simulink model "VirtualDAQ"  (R2021b)
settings: Solver=VariableStepAuto  StartTime=0.0  StopTime=inf  MaxStep=0.001  RelTol=1e-3
libraries: fl_lib x5, simulink x3, nesl_utility x3, dspxfrm3 x1
(part 2 of 2)

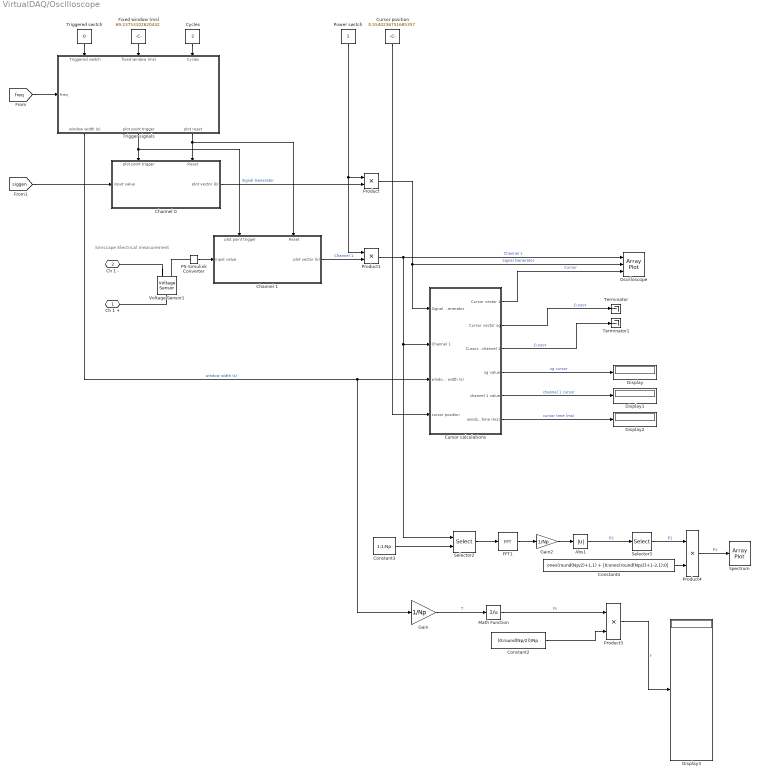
== system VirtualDAQ/Oscilloscope ==
  note: Simscape Electrical measurement
  Abs1 : Abs
  Channel 0 : Subsystem
      settings: PortSchema="{\"entries\":[{\"content\":{\"sides\":[{\"content\":{\"connectorIds\":[\"In1\"]},\"type\":\"ConnectorPlacement.EquallySpacedRectSide\",\"uuid\":\"56eea059-d5e9-4d95-b7d9-83a317b3103e\"},{\"content\":{\"connectorIds\":[\"Out1\"],\"side\":\"RIGHT\"},\"type\":\"ConnectorPlacement.EquallySpacedRectSide\",\"uuid\":\"fd8b8cd5-6def-4d8f-87ca-646372cc7fbe\"},{\"content\":{\"connectorIds\":[\"In2\",\"In3\"],\"side\":\"TOP\"},\"type\":\"ConnectorPlacement.EquallySpacedRectSide\",\"uuid\":\"3d9c38ee-b24b-466c-a7ac-a6d8a7456d51\"},{\"content\":{\"connectorIds\":[],\"side\":\"BOTTOM\"},\"type\":\"ConnectorPlacement.EquallySpacedRectSide\",\"uuid\":\"336136fa-2514-49ab-9e17-88caaca7366c\"}]},\"type\":\"ConnectorPlacement.EquallySpacedConnector\",\"uuid\":\"1d9824a8-6efd-49ff-b082-cf2ede19b4fd\"}],\"packageUris\":[\"http://schema.mathworks.com/mf0/Connector/R2020b\"],\"version\":\"1.0\"}"
  Channel 1 : Subsystem
      settings: PortSchema="{\"entries\":[{\"content\":{\"sides\":[{\"content\":{\"connectorIds\":[\"In1\"]},\"type\":\"ConnectorPlacement.EquallySpacedRectSide\",\"uuid\":\"56eea059-d5e9-4d95-b7d9-83a317b3103e\"},{\"content\":{\"connectorIds\":[\"Out1\"],\"side\":\"RIGHT\"},\"type\":\"ConnectorPlacement.EquallySpacedRectSide\",\"uuid\":\"fd8b8cd5-6def-4d8f-87ca-646372cc7fbe\"},{\"content\":{\"connectorIds\":[\"In2\",\"In3\"],\"side\":\"TOP\"},\"type\":\"ConnectorPlacement.EquallySpacedRectSide\",\"uuid\":\"3d9c38ee-b24b-466c-a7ac-a6d8a7456d51\"},{\"content\":{\"connectorIds\":[],\"side\":\"BOTTOM\"},\"type\":\"ConnectorPlacement.EquallySpacedRectSide\",\"uuid\":\"336136fa-2514-49ab-9e17-88caaca7366c\"}]},\"type\":\"ConnectorPlacement.EquallySpacedConnector\",\"uuid\":\"1d9824a8-6efd-49ff-b082-cf2ede19b4fd\"}],\"packageUris\":[\"http://schema.mathworks.com/mf0/Connector/R2020b\"],\"version\":\"1.0\"}"
  Constant2 : Constant  Value=(0:round(Np/2))/Np
  Constant3 : Constant  Value=1:1:Np
  Constant4 : Constant  Value=ones(round(Np/2)+1,1) + [0;ones(round(Np/2)+1-2,1);0]
  Cursor calculations : Subsystem
  Cursor position : Constant  Value=0.5540236751685357
  Cycles : Constant  Value=2
  Display{,1..3} (4 alike) : Display
  FFT1 : dspxfrm3/FFT  FFTImplementation=Auto  CompMethod=Table lookup  TableOpt=NEW  TableOptActive=Speed  BitRevOrder=off  Normalize=off  InheritFFTLength=on  FFTLength=64  WrapInput=on  roundingMode=Floor  overflowMode=off  firstCoeffDataTypeStr=Inherit: Same word length as input  firstCoeffLastDataTypeStr=Inherit: Same word length as input  outputMin=[]  outputMax=[]
  Fixed window (ms) : Constant  Value=69.23753102620442
  Gain : Gain  Gain=1/Np
  Gain2 : Gain  Gain=1/Np
  Math Function : Math  Operator=reciprocal  SaturateOnIntegerOverflow=on
  Oscilloscope : ArrayPlot  NumInputPorts=3  WindowPosition=[1282.000000,742.000000,1279.000000,669.000000,]  Visible=on  PlotType=Line  AxesScaling=Manual  YLimits=[-5.1,5.1]  ShowLegend=on
  PS-Simulink Converter : nesl_utility/PS-Simulink Converter  PhysicalDomain=network_engine_domain  SubClassName=ps_output  LeftPortType=input  RightPortType=output  PseudoPeriodic=off  Frequencies=[]  Unit=inherit  AffineConversion=off
      settings: SourceProductBaseCode=PW,SS
  Power switch : Constant
  Product{,1,3..4} (4 alike) : Product
  Selector2 : Selector  InputPortWidth=Np  IndexOptions=Index vector (port)  Indices=1:4:Np  OutputSizes=1
  Selector3 : Selector  InputPortWidth=Np  IndexOptions=Index vector (dialog)  Indices=1:round(Np/2)+1  OutputSizes=1
  Spectrum : ArrayPlot  WindowPosition=[1282.000000,42.000000,1279.000000,669.000000,]  Visible=on  YLimits=[-0.20978091343649902,1.9504387414806172]
  Terminator : Terminator
  Terminator1 : Terminator
  Trigger signals : Subsystem
      settings: PortSchema="{\"entries\":[{\"content\":{\"sides\":[{\"content\":{\"connectorIds\":[\"In1\"]},\"type\":\"ConnectorPlacement.EquallySpacedRectSide\",\"uuid\":\"b92255b7-066e-487b-9e0c-e19692fc940f\"},{\"content\":{\"connectorIds\":[],\"side\":\"RIGHT\"},\"type\":\"ConnectorPlacement.EquallySpacedRectSide\",\"uuid\":\"cb964d42-f40b-466c-b45b-853437324272\"},{\"content\":{\"connectorIds\":[\"In2\",\"In3\",\"In4\"],\"side\":\"TOP\"},\"type\":\"ConnectorPlacement.EquallySpacedRectSide\",\"uuid\":\"e1027385-b295-47a3-ae7d-2e3bb07fa1de\"},{\"content\":{\"connectorIds\":[\"Out1\",\"Out2\",\"Out3\"],\"side\":\"BOTTOM\"},\"type\":\"ConnectorPlacement.EquallySpacedRectSide\",\"uuid\":\"c27dc584-c0ba-4e72-b8bf-7374d1985911\"}]},\"type\":\"ConnectorPlacement.EquallySpacedConnector\",\"uuid\":\"1db11e79-2cf0-4841-86d9-651820ebc8ee\"}],\"packageUris\":[\"http://schema.mathworks.com/mf0/Connector/R2020b\"],\"version\":\"1.0\"}"
  Triggered switch : Constant  Value=0
  Voltage Sensor1 : fl_lib/Electrical/Electrical Sensors/Voltage Sensor
  Ch 1 + : PMIOPort  Side=Right
  Ch 1 - : PMIOPort  Port=2  Side=Right
  wires:
  PS-Simulink Converter/1 -> Channel 1/1(input value)
  Trigger signals/3("plot reset ") -> Channel 0/3(Reset), Channel 1/3(Reset)
  Trigger signals/2(plot point trigger) -> Channel 0/2(plot point trigger), Channel 1/2(plot point trigger)
  [freq] -> Trigger signals/1(freq)
  Product/1 -> Oscilloscope/2, Cursor calculations/1(Signal Generator)  "Signal Generator"
  [siggen] -> Channel 0/1(input value)
  Power switch/1 -> Product1/1, Product/1
  Channel 0/1(plot vector (k)) -> Product/2  "Signal Generator"
  Channel 1/1(plot vector (k)) -> Product1/2  "Channel 1"
  Triggered switch/1 -> Trigger signals/2(Triggered switch)
  Cycles/1 -> Trigger signals/4(Cycles)
  Cursor position/1 -> Cursor calculations/4(cursor position)
  Cursor calculations/1(Cursor vector 1) -> Oscilloscope/3  "Cursor"
  Cursor calculations/4(sg value) -> Display/1  "sg cursor"
  Cursor calculations/5(channel 1 value) -> Display1/1  "channel 1 cursor"
  Cursor calculations/3(Cursor vector channel 1) -> Terminator1/1  "Cursor"
  Cursor calculations/6(window time (ms)) -> Display2/1  "cursor time (ms)"
  Cursor calculations/2(Cursor vector sg) -> Terminator/1  "Cursor"
  Trigger signals/1(window width (s)) -> Gain/1, Cursor calculations/3(window width (s))  "window width (s)"
  Fixed window (ms)/1 -> Trigger signals/3(fixed window (ms))
  Gain/1 -> Math Function/1  "T"
  Math Function/1 -> Product3/1  "Fs"
  Constant2/1 -> Product3/2
  Product3/1 -> Display3/1  "f"
  Constant4/1 -> Product4/2
  FFT1/1 -> Gain2/1
  Constant3/1 -> Selector2/2
  Product4/1 -> Spectrum/1  "P1"
  Product1/1 -> Cursor calculations/2(Channel 1), Selector2/1, Oscilloscope/1  "Channel 1"
  Selector2/1 -> FFT1/1
  Gain2/1 -> Abs1/1
  Selector3/1 -> Product4/1  "P1"
  Abs1/1 -> Selector3/1  "P2"
  connections:
  Voltage Sensor1/RConn2 -- Ch 1 -/RConn1
  Voltage Sensor1/RConn1 -- PS-Simulink Converter/LConn1
  Voltage Sensor1/LConn1 -- Ch 1 +/RConn1

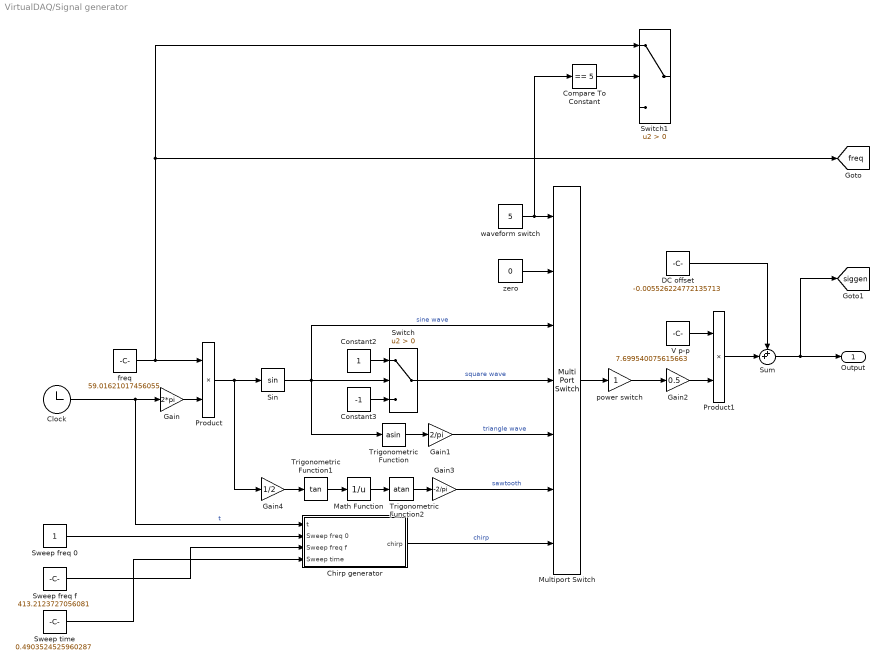
== system VirtualDAQ/Signal generator ==
  Chirp generator : Subsystem
  Clock : Clock
  Compare To Constant : simulink/Logic and Bit Operations/Compare To Constant  relop===  const=5  OutDataTypeStr=boolean
  Constant2 : Constant  SampleTime=0
  Constant3 : Constant  Value=-1  SampleTime=0
  DC offset : Constant  Value=-0.005526224772135713
  Gain : Gain  Gain=2*pi
  Gain1 : Gain  Gain=2/pi
  Gain2 : Gain  Gain=0.5
  Gain3 : Gain  Gain=-2/pi
  Gain4 : Gain  Gain=1/2
  Math Function : Math  Operator=reciprocal  SaturateOnIntegerOverflow=on
  Multiport Switch : MultiPortSwitch  DataPortOrder=Zero-based contiguous  Inputs=6  DiagnosticForDefault=None  zeroidx=on
  Product : Product
  Product1 : Product
  Sin : Trigonometry
  Sum : Sum  Inputs=++|
  Sweep freq 0 : Constant
  Sweep freq f : Constant  Value=413.2123727056081
  Sweep time : Constant  Value=0.4903524525960287
  Switch : Switch  Criteria=u2 > Threshold
  Switch1 : Switch  Criteria=u2 > Threshold
  Trigonometric Function : Trigonometry  Operator=asin
  Trigonometric Function1 : Trigonometry  Operator=tan
  Trigonometric Function2 : Trigonometry  Operator=atan
  V p-p : Constant  Value=7.699540075615663  SampleTime=-1
  freq : Constant  Value=59.01621017456055  SampleTime=0
  power switch : Gain
  waveform switch : Constant  Value=5  SampleTime=0
  zero : Constant  Value=0  SampleTime=0
  Output : Outport
  tag scope: freq=global, siggen=global
  wires:
  Sin/1 -> Trigonometric Function/1, Multiport Switch/3, Switch/2  "sine wave"
  freq/1 -> Switch1/1, [freq], Product/1
  Clock/1 -> Chirp generator/1(t), Gain/1  "t"
  power switch/1 -> Gain2/1
  zero/1 -> Multiport Switch/2
  Trigonometric Function/1 -> Gain1/1
  Constant2/1 -> Switch/1
  Constant3/1 -> Switch/3
  Gain2/1 -> Product1/2
  Product/1 -> Sin/1, Gain4/1
  Gain1/1 -> Multiport Switch/5  "triangle wave"
  Math Function/1 -> Trigonometric Function2/1
  Trigonometric Function1/1 -> Math Function/1
  Trigonometric Function2/1 -> Gain3/1
  Gain4/1 -> Trigonometric Function1/1
  Multiport Switch/1 -> power switch/1
  Gain3/1 -> Multiport Switch/6  "sawtooth"
  V p-p/1 -> Product1/1
  Product1/1 -> Sum/2
  DC offset/1 -> Sum/1
  Switch/1 -> Multiport Switch/4  "square wave"
  Sum/1 -> [siggen], Output/1
  Gain/1 -> Product/2
  Sweep time/1 -> Chirp generator/4(Sweep time)
  Chirp generator/1(chirp) -> Multiport Switch/7  "chirp"
  Sweep freq 0/1 -> Chirp generator/2(Sweep freq 0)
  Sweep freq f/1 -> Chirp generator/3(Sweep freq f)
  Compare To Constant/1 -> Switch1/2
  waveform switch/1 -> Compare To Constant/1, Multiport Switch/1

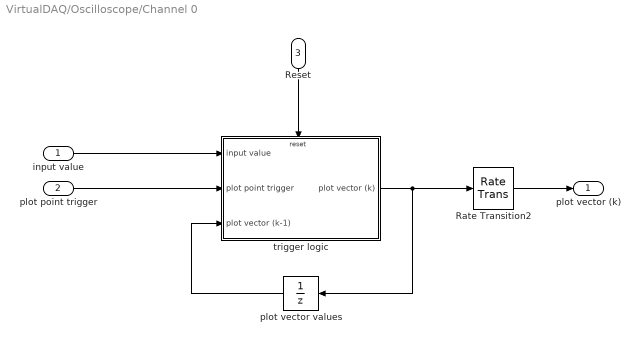
== system VirtualDAQ/Oscilloscope/Channel 0 ==
  input value : Inport
  plot point trigger : Inport  Port=2
  Reset : Inport  Port=3
  Rate Transition2 : RateTransition  InitialCondition=zeros(Np,1)  OutPortSampleTime=1/refreshRate
  plot vector values : UnitDelay  InitialCondition=zeros(Np,1)  SampleTime=-1  HasFrameUpgradeWarning=on
  trigger logic : Subsystem  TreatAsAtomicUnit=on
  plot vector (k) : Outport
  wires:
  plot vector values/1 -> trigger logic/3(plot vector (k-1))
  plot point trigger/1 -> trigger logic/2(plot point trigger)
  trigger logic/1(plot vector (k)) -> Rate Transition2/1, plot vector values/1
  Reset/1 -> trigger logic/Reset
  input value/1 -> trigger logic/1(input value)
  Rate Transition2/1 -> plot vector (k)/1

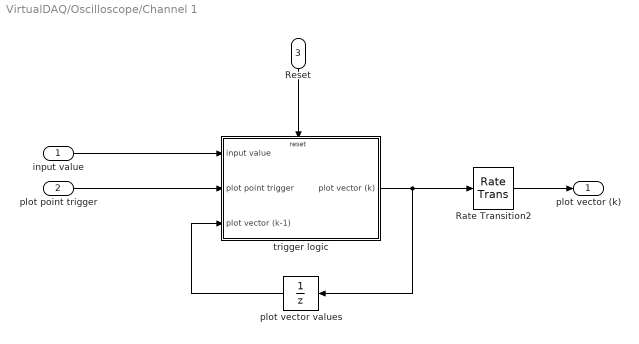
== system VirtualDAQ/Oscilloscope/Channel 1 ==
  input value : Inport
  plot point trigger : Inport  Port=2
  Reset : Inport  Port=3
  Rate Transition2 : RateTransition  InitialCondition=zeros(Np,1)  OutPortSampleTime=1/refreshRate
  plot vector values : UnitDelay  InitialCondition=zeros(Np,1)  SampleTime=-1  HasFrameUpgradeWarning=on
  trigger logic : Subsystem  TreatAsAtomicUnit=on
  plot vector (k) : Outport
  wires:
  plot vector values/1 -> trigger logic/3(plot vector (k-1))
  plot point trigger/1 -> trigger logic/2(plot point trigger)
  trigger logic/1(plot vector (k)) -> Rate Transition2/1, plot vector values/1
  Reset/1 -> trigger logic/Reset
  input value/1 -> trigger logic/1(input value)
  Rate Transition2/1 -> plot vector (k)/1

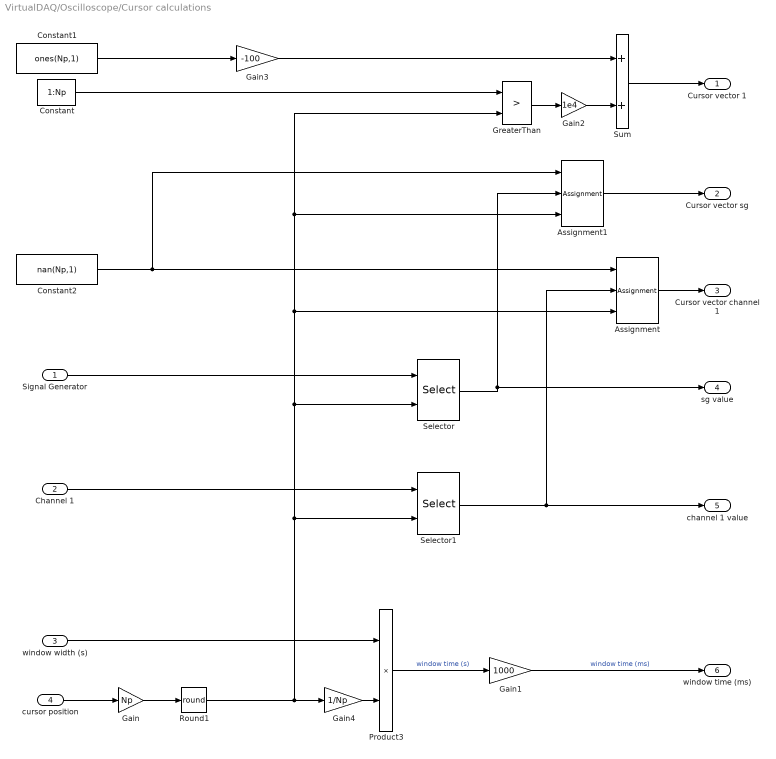
== system VirtualDAQ/Oscilloscope/Cursor calculations ==
  Signal Generator : Inport
  Channel 1 : Inport  Port=2
  window width (s) : Inport  Port=3
  cursor position : Inport  Port=4
  Assignment : Assignment  DiagnosticForDimensions=Warning  IndexOptions=Index vector (port)  Indices=1  OutputSizes=1
  Assignment1 : Assignment  DiagnosticForDimensions=Warning  IndexOptions=Index vector (port)  Indices=1  OutputSizes=1
  Constant : Constant  Value=1:Np
  Constant1 : Constant  Value=ones(Np,1)
  Constant2 : Constant  Value=nan(Np,1)
  Gain : Gain  Gain=Np
  Gain1 : Gain  Gain=1000
  Gain2 : Gain  Gain=1e4
  Gain3 : Gain  Gain=-100
  Gain4 : Gain  Gain=1/Np
  GreaterThan : RelationalOperator  Operator=>  OutDataTypeStr=boolean  RndMeth=Simplest
  Product3 : Product
  Round1 : Rounding  Operator=round
  Selector : Selector  InputPortWidth=Np  IndexOptions=Index vector (port)  Indices=[1 3]  OutputSizes=1
  Selector1 : Selector  InputPortWidth=Np  IndexOptions=Index vector (port)  Indices=[1 3]  OutputSizes=1
  Sum : Sum
  Cursor vector 1 : Outport
  Cursor vector sg : Outport  Port=2
  Cursor vector channel 1 : Outport  Port=3
  sg value : Outport  Port=4
  channel 1 value : Outport  Port=5
  window time (ms) : Outport  Port=6
  wires:
  cursor position/1 -> Gain/1
  Constant/1 -> GreaterThan/1
  Product3/1 -> Gain1/1  "window time (s)"
  Gain1/1 -> window time (ms)/1  "window time (ms)"
  GreaterThan/1 -> Gain2/1
  Sum/1 -> Cursor vector 1/1
  Gain2/1 -> Sum/2
  Signal Generator/1 -> Selector/1
  Selector1/1 -> Assignment/2, channel 1 value/1
  Constant1/1 -> Gain3/1
  Gain3/1 -> Sum/1
  Gain/1 -> Round1/1
  Gain4/1 -> Product3/2
  Channel 1/1 -> Selector1/1
  Assignment/1 -> Cursor vector channel 1/1
  Selector/1 -> Assignment1/2, sg value/1
  Round1/1 -> Selector/2, Assignment1/3, GreaterThan/2, Assignment/3, Selector1/2, Gain4/1
  Assignment1/1 -> Cursor vector sg/1
  Constant2/1 -> Assignment1/1, Assignment/1
  window width (s)/1 -> Product3/1

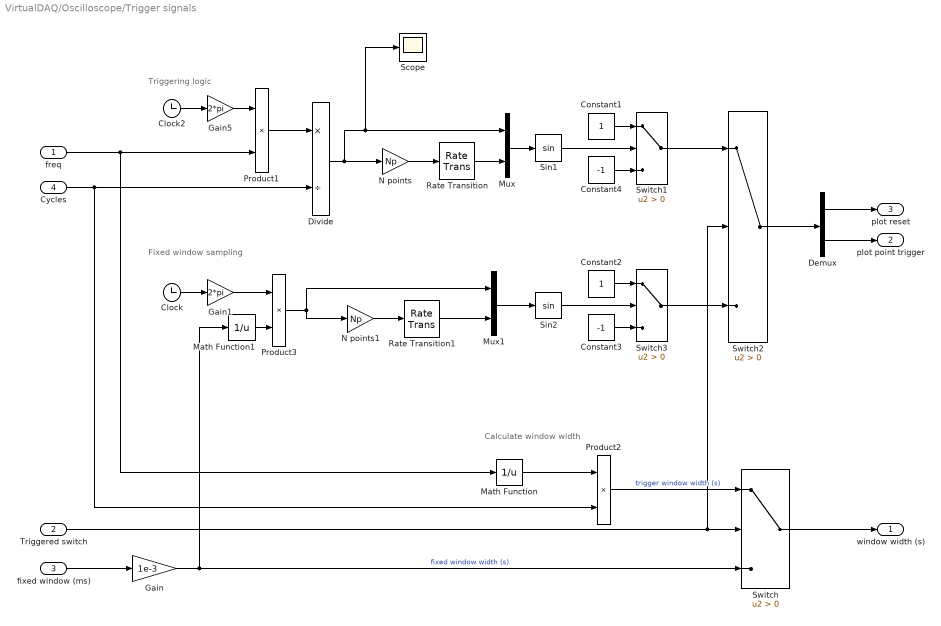
== system VirtualDAQ/Oscilloscope/Trigger signals ==
  note: Calculate window width
  note: Triggering logic
  note: Fixed window sampling
  freq : Inport
  Triggered switch : Inport  Port=2
  fixed window (ms) : Inport  Port=3
  Cycles : Inport  Port=4
  Clock : Clock
  Clock2 : Clock
  Constant1 : Constant  SampleTime=0
  Constant2 : Constant  SampleTime=0
  Constant3 : Constant  Value=-1  SampleTime=0
  Constant4 : Constant  Value=-1  SampleTime=0
  Demux : Demux  Outputs=2
  Divide : Product  Inputs=*/
  Gain : Gain  Gain=1e-3
  Gain1 : Gain  Gain=2*pi
  Gain5 : Gain  Gain=2*pi
  Math Function : Math  Operator=reciprocal  SaturateOnIntegerOverflow=on
  Math Function1 : Math  Operator=reciprocal  SaturateOnIntegerOverflow=on
  Mux : Mux  Inputs=2
  Mux1 : Mux  Inputs=2
  N points : Gain  Gain=Np
  N points1 : Gain  Gain=Np
  Product1 : Product
  Product2 : Product
  Product3 : Product
  Rate Transition : RateTransition  OutPortSampleTime=plot_dt
  Rate Transition1 : RateTransition  OutPortSampleTime=plot_dt
  Scope : Scope
  Sin1 : Trigonometry
  Sin2 : Trigonometry
  Switch{,1..3} (4 alike) : Switch  Criteria=u2 > Threshold
  window width (s) : Outport
  plot point trigger : Outport  Port=2
  "plot reset " : Outport  Port=3
  wires:
  Gain5/1 -> Product1/1
  Constant4/1 -> Switch1/3
  Clock2/1 -> Gain5/1
  Sin1/1 -> Switch1/2
  Constant1/1 -> Switch1/1
  Product1/1 -> Divide/1
  Divide/1 -> Scope/1, Mux/1, N points/1
  N points/1 -> Rate Transition/1
  Mux/1 -> Sin1/1
  Demux/2 -> plot point trigger/1
  Demux/1 -> "plot reset "/1
  Rate Transition/1 -> Mux/2
  Triggered switch/1 -> Switch/2, Switch2/2
  Product2/1 -> Switch/1  "trigger window width (s)"
  freq/1 -> Product1/2, Math Function/1
  Cycles/1 -> Divide/2, Product2/2
  Math Function/1 -> Product2/1
  fixed window (ms)/1 -> Gain/1
  Switch/1 -> window width (s)/1
  Switch1/1 -> Switch2/1
  Switch2/1 -> Demux/1
  N points1/1 -> Rate Transition1/1
  Rate Transition1/1 -> Mux1/2
  Constant2/1 -> Switch3/1
  Sin2/1 -> Switch3/2
  Constant3/1 -> Switch3/3
  Switch3/1 -> Switch2/3
  Mux1/1 -> Sin2/1
  Clock/1 -> Gain1/1
  Product3/1 -> Mux1/1, N points1/1
  Gain/1 -> Switch/3, Math Function1/1  "fixed window width (s)"
  Gain1/1 -> Product3/1
  Math Function1/1 -> Product3/2

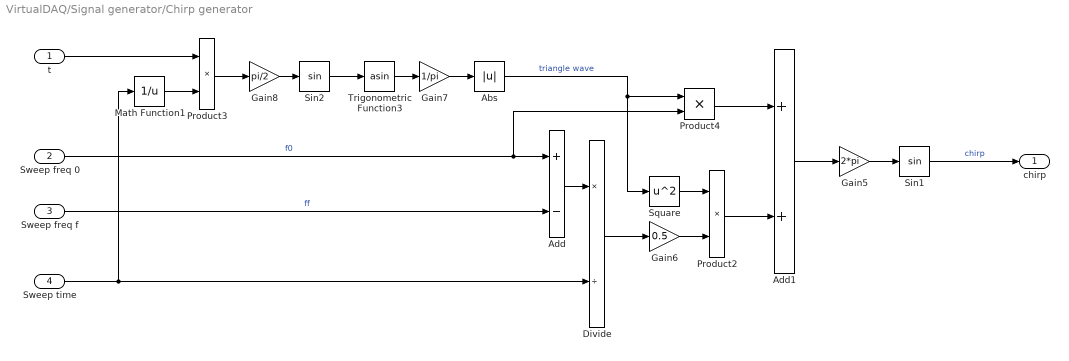
== system VirtualDAQ/Signal generator/Chirp generator ==
  t : Inport
  Sweep freq 0 : Inport  Port=2
  Sweep freq f : Inport  Port=3
  Sweep time : Inport  Port=4
  Abs : Abs
  Add : Sum  Inputs=+-
  Add1 : Sum
  Divide : Product  Inputs=*/
  Gain5 : Gain  Gain=2*pi
  Gain6 : Gain  Gain=0.5
  Gain7 : Gain  Gain=1/pi
  Gain8 : Gain  Gain=pi/2
  Math Function1 : Math  Operator=reciprocal  SaturateOnIntegerOverflow=on
  Product2 : Product
  Product3 : Product
  Product4 : Product
  Sin1 : Trigonometry
  Sin2 : Trigonometry
  Square : Math  Operator=square  SaturateOnIntegerOverflow=on
  Trigonometric Function3 : Trigonometry  Operator=asin
  chirp : Outport
  wires:
  Add/1 -> Divide/1
  Add1/1 -> Gain5/1
  Abs/1 -> Square/1, Product4/1  "triangle wave"
  Gain5/1 -> Sin1/1
  Gain8/1 -> Sin2/1
  Divide/1 -> Gain6/1
  Product4/1 -> Add1/1
  Gain6/1 -> Product2/2
  Product2/1 -> Add1/2
  Square/1 -> Product2/1
  Sweep time/1 -> Divide/2, Math Function1/1
  Gain7/1 -> Abs/1
  t/1 -> Product3/1
  Sin2/1 -> Trigonometric Function3/1
  Trigonometric Function3/1 -> Gain7/1
  Math Function1/1 -> Product3/2
  Product3/1 -> Gain8/1
  Sin1/1 -> chirp/1  "chirp"
  Sweep freq 0/1 -> Product4/2, Add/1  "f0"
  Sweep freq f/1 -> Add/2  "ff"

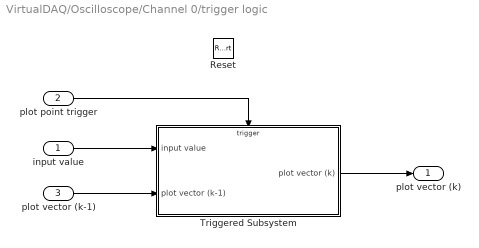
== system VirtualDAQ/Oscilloscope/Channel 0/trigger logic ==
  input value : Inport
  plot point trigger : Inport  Port=2
  plot vector (k-1) : Inport  Port=3
  Reset : ResetPort  DisableCoverage=on
  Triggered Subsystem : Subsystem  TreatAsAtomicUnit=on
  plot vector (k) : Outport
  wires:
  plot point trigger/1 -> Triggered Subsystem/Trigger
  input value/1 -> Triggered Subsystem/1(input value)
  Triggered Subsystem/1(plot vector (k)) -> plot vector (k)/1
  plot vector (k-1)/1 -> Triggered Subsystem/2(plot vector (k-1))

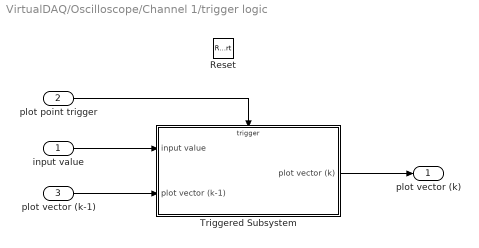
== system VirtualDAQ/Oscilloscope/Channel 1/trigger logic ==
  input value : Inport
  plot point trigger : Inport  Port=2
  plot vector (k-1) : Inport  Port=3
  Reset : ResetPort  DisableCoverage=on
  Triggered Subsystem : Subsystem  TreatAsAtomicUnit=on
  plot vector (k) : Outport
  wires:
  plot point trigger/1 -> Triggered Subsystem/Trigger
  input value/1 -> Triggered Subsystem/1(input value)
  Triggered Subsystem/1(plot vector (k)) -> plot vector (k)/1
  plot vector (k-1)/1 -> Triggered Subsystem/2(plot vector (k-1))

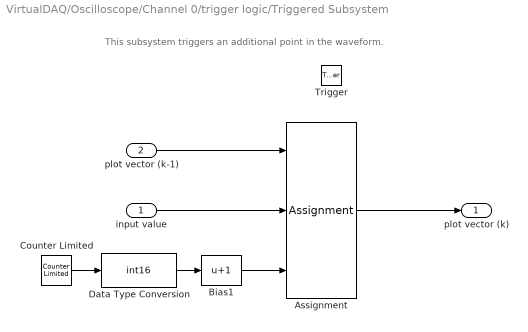
== system VirtualDAQ/Oscilloscope/Channel 0/trigger logic/Triggered Subsystem ==
  note: This subsystem triggers an additional point in the waveform.
  input value : Inport
  plot vector (k-1) : Inport  Port=2
  Trigger : TriggerPort  VariantControl=(inherit)
  Assignment : Assignment  DiagnosticForDimensions=Warning  IndexOptions=Index vector (port)  Indices=1  OutputSizes=1
  Bias1 : Bias  Bias=1
  Counter Limited : simulink/Sources/Counter Limited  uplimit=Np-1  tsamp=-1
  Data Type Conversion : DataTypeConversion  OutDataTypeStr=int16
  plot vector (k) : Outport
  wires:
  Assignment/1 -> plot vector (k)/1
  input value/1 -> Assignment/2
  Counter Limited/1 -> Data Type Conversion/1
  Bias1/1 -> Assignment/3
  plot vector (k-1)/1 -> Assignment/1
  Data Type Conversion/1 -> Bias1/1

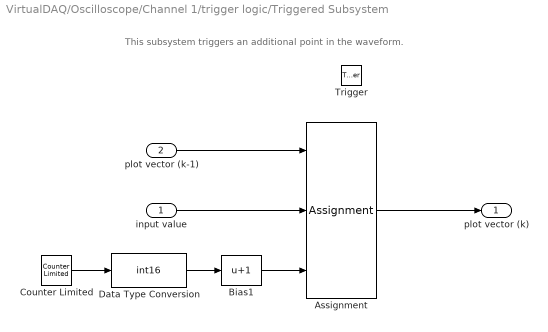
== system VirtualDAQ/Oscilloscope/Channel 1/trigger logic/Triggered Subsystem ==
  note: This subsystem triggers an additional point in the waveform.
  input value : Inport
  plot vector (k-1) : Inport  Port=2
  Trigger : TriggerPort  VariantControl=(inherit)
  Assignment : Assignment  DiagnosticForDimensions=Warning  IndexOptions=Index vector (port)  Indices=1  OutputSizes=1
  Bias1 : Bias  Bias=1
  Counter Limited : simulink/Sources/Counter Limited  uplimit=Np-1  tsamp=-1
  Data Type Conversion : DataTypeConversion  OutDataTypeStr=int16
  plot vector (k) : Outport
  wires:
  Assignment/1 -> plot vector (k)/1
  input value/1 -> Assignment/2
  Counter Limited/1 -> Data Type Conversion/1
  Bias1/1 -> Assignment/3
  plot vector (k-1)/1 -> Assignment/1
  Data Type Conversion/1 -> Bias1/1
